simulink model "Joystick_Controller"  (R2025b)
settings: Solver=VariableStepAuto  StartTime=0.0  StopTime=inf  RelTol=1e-3
undefined symbols (not defined in the file): battery_voltage, force_table, pwm_list, voltage_list
libraries: ros2lib x3
settings Model: Creator=vulcangrip  LastModifiedBy=vulcangrip

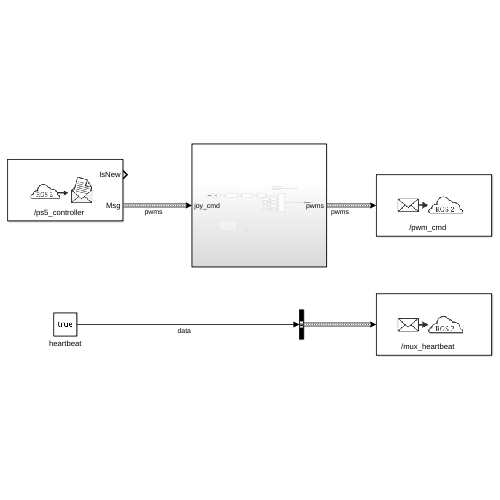
[thumbnail: Simulink's stored preview of the top-level diagram]
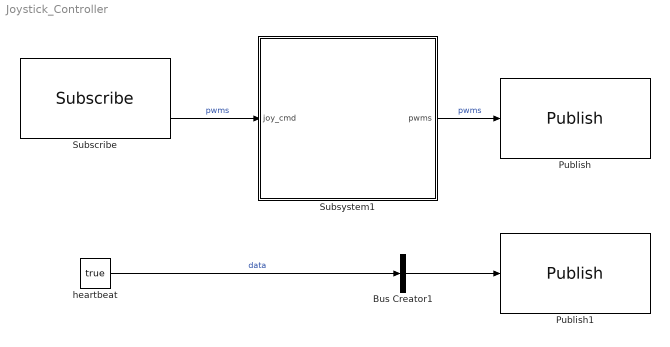
== system Joystick_Controller ==
  Bus Creator1 : BusCreator  Inputs=1  OutDataTypeStr=Bus: SL_Bus_std_msgs_Bool  NonVirtualBus=on
  Publish : ros2lib/Publish  topicSource=Specify your own  topic=/pwm_cmd  messageType=custom_interfaces/Pwms  QOSHistory=Keep last  QOSDepth=10  QOSReliability=Reliable  QOSDurability=Volatile  QOSDeadline=Inf  QOSLifespan=Inf  QOSLiveliness=Automatic  QOSLeaseDuration=Inf  QOSAvoidROSNamespaceConventions=off
  Publish1 : ros2lib/Publish  topicSource=Specify your own  topic=/mux_heartbeat  messageType=std_msgs/Bool  QOSHistory=Keep last  QOSDepth=10  QOSReliability=Reliable  QOSDurability=Volatile  QOSDeadline=Inf  QOSLifespan=Inf  QOSLiveliness=Automatic  QOSLeaseDuration=Inf  QOSAvoidROSNamespaceConventions=off
  Subscribe : ros2lib/Subscribe  topicSource=Specify your own  topic=/ps5_controller  messageType=remote_control_interface/Gamepad  sampleTime=1/60  QOSHistory=Keep last  QOSDepth=10  QOSReliability=Reliable  QOSDurability=Volatile  QOSDeadline=Inf  QOSLifespan=Inf  QOSLiveliness=Automatic  QOSLeaseDuration=Inf  QOSAvoidROSNamespaceConventions=off
  Subsystem1 : Subsystem
  heartbeat : Constant  Value=true
  wires:
  Bus Creator1/1 -> Publish1/1
  heartbeat/1 -> Bus Creator1/1  "data"
  Subscribe/2 -> Subsystem1/1(joy_cmd)  "pwms"
  Subsystem1/1(pwms) -> Publish/1  "pwms"

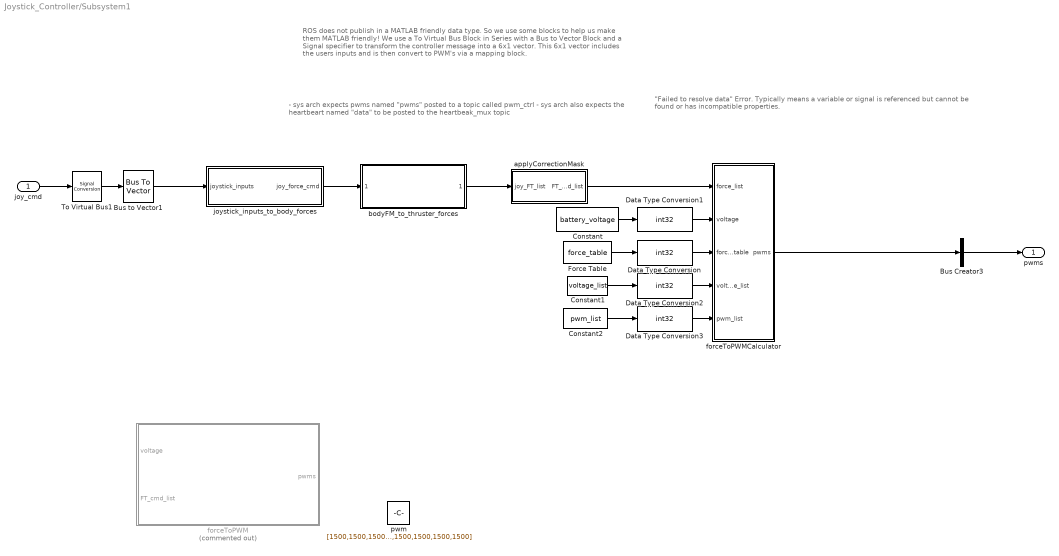
== system Joystick_Controller/Subsystem1 ==
  note: "Failed to resolve data" Error.
      |
      | Typically means a variable or signal is referenced but cannot be found or has incompatible properties.
  note: ROS does not publish in a MATLAB friendly data type. So we use some blocks to help us make them MATLAB friendly!
      |
      | We use a To Virtual Bus Block in Series with a Bus to Vector Block and a Signal specifier to transform the controller message into a 6x1 vector. This 6x1 vector includes the users inputs and is then convert to PWM's via a mapping block.
  note: - sys arch expects pwms named "pwms" posted to a topic called pwm_ctrl
      | - sys arch also expects the heartbeart  named "data" to be posted to the heartbeak_mux topic
  joy_cmd : Inport
  Bus Creator3 : BusCreator  Inputs=1  OutDataTypeStr=Bus: SL_Bus_custom_interfaces_Pwms  NonVirtualBus=on
  Bus to Vector1 : BusToVector
  Constant : Constant  Value=battery_voltage  OutDataTypeStr=int32
  Constant1 : Constant  Value=voltage_list  OutDataTypeStr=int32
  Constant2 : Constant  Value=pwm_list  OutDataTypeStr=int32
  Data Type Conversion{,1..3} (4 alike) : DataTypeConversion  OutDataTypeStr=int32  SaturateOnIntegerOverflow=off  RndMeth=Floor
  Force Table : Constant  Value=force_table  OutDataTypeStr=int32
  To Virtual Bus1 : SignalConversion  ConversionOutput=Virtual bus  OverrideOpt=off
  applyCorrectionMask : Subsystem
  bodyFM_to_thruster_forces : Subsystem  ReferencedSubsystem=bodyFM_to_thruster_forces
  forceToPWM : Subsystem  Commented=on
  forceToPWMCalculator : MATLAB Function  TreatAsAtomicUnit=on
  joystick_inputs_to_body_forces : MATLAB Function  TreatAsAtomicUnit=on
  pwm : Constant  Value=[1500,1500,1500,1500,1500,1500,1500,1500]  OutDataTypeStr=int32
  pwms : Outport
  wires:
  joy_cmd/1 -> To Virtual Bus1/1
  To Virtual Bus1/1 -> Bus to Vector1/1
  Bus to Vector1/1 -> joystick_inputs_to_body_forces/1(joystick_inputs)
  joystick_inputs_to_body_forces/1(joy_force_cmd) -> bodyFM_to_thruster_forces/1
  Bus Creator3/1 -> pwms/1
  bodyFM_to_thruster_forces/1 -> applyCorrectionMask/1(joy_FT_list)
  Constant2/1 -> Data Type Conversion3/1
  Constant/1 -> Data Type Conversion1/1
  Force Table/1 -> Data Type Conversion/1
  Constant1/1 -> Data Type Conversion2/1
  forceToPWMCalculator/1(pwms) -> Bus Creator3/1
  applyCorrectionMask/1(FT_cmd_list) -> forceToPWMCalculator/1(force_list)
  Data Type Conversion1/1 -> forceToPWMCalculator/2(voltage)
  Data Type Conversion/1 -> forceToPWMCalculator/3(force_table)
  Data Type Conversion2/1 -> forceToPWMCalculator/4(voltage_list)
  Data Type Conversion3/1 -> forceToPWMCalculator/5(pwm_list)

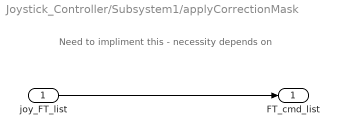
== system Joystick_Controller/Subsystem1/applyCorrectionMask ==
  note: Need to impliment this - necessity depends on
  joy_FT_list : Inport
  FT_cmd_list : Outport
  wires:
  joy_FT_list/1 -> FT_cmd_list/1

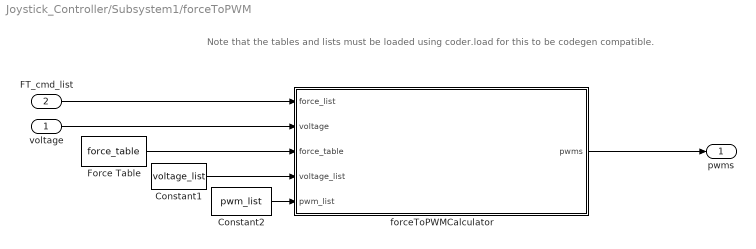
== system Joystick_Controller/Subsystem1/forceToPWM ==
  note: Note that the tables and lists must be loaded using coder.load for this to be codegen compatible.
  voltage : Inport
  FT_cmd_list : Inport  Port=2
  Constant1 : Constant  Value=voltage_list
  Constant2 : Constant  Value=pwm_list
  Force Table : Constant  Value=force_table
  forceToPWMCalculator : MATLAB Function  TreatAsAtomicUnit=on
  pwms : Outport
  wires:
  voltage/1 -> forceToPWMCalculator/2(voltage)
  Constant1/1 -> forceToPWMCalculator/4(voltage_list)
  Constant2/1 -> forceToPWMCalculator/5(pwm_list)
  Force Table/1 -> forceToPWMCalculator/3(force_table)
  FT_cmd_list/1 -> forceToPWMCalculator/1(force_list)
  forceToPWMCalculator/1(pwms) -> pwms/1

== matlab function Joystick_Controller/Subsystem1/forceToPWM/forceToPWMCalculator ==
  data: force_list input; voltage input; pwms output; force_table input; voltage_list input; pwm_list input
function pwms = fcn(force_list,voltage,force_table,voltage_list,pwm_list)

pwms = int32([1500,1500,1500,1500,1500,1500,1500,1500]);

== matlab function Joystick_Controller/Subsystem1/forceToPWMCalculator ==
  data: force_list input; voltage input; pwms output; force_table input; voltage_list input; pwm_list input
function pwms = forceToPWMCalculator(force_list,voltage,force_table,voltage_list,pwm_list)

%pwms = int32(force_list*battery_voltage);
%{
This function figures out what pwm to send in order to get the appropriate
force at the current voltage.


%}
pwms = int32(zeros(size(force_list)));

for k = 1:length(force_list)
    force = force_list(k);

    if(abs(force)<1e-3)
        %if the force setting is very low, just set thruster to stop
        %condition
        pwm_cmd = int32(1500);
    else
        
        %find the closest voltage less than the input voltage
        [~,closest_index] = min(abs(voltage_list-voltage));
       
        %see if the closest_voltage is above or below the input voltage
        if(closest_index==int32(1))
            %no need to do any interpolation, just take the first column for forces
            lower_voltage_index = int32(1);
            upper_voltage_index = int32(1);
    
        elseif(closest_index==length(voltage_list))
            %no need to do any interpolation, just take the last column for forces
            lower_voltage_index = int32(length(voltage_list));
            upper_voltage_index = int32(length(voltage_list));
        elseif(voltage_list(closest_index) < voltage)
            lower_voltage_index = int32(closest_index);
            upper_voltage_index = int32(closest_index+1);
        else
            upper_voltage_index = int32(closest_index);
            lower_voltage_index = int32(closest_index-1);
        end
        
        %average the force column between the two indices\
        if(upper_voltage_index == lower_voltage_index)
            force_column = force_table(lower_voltage_index);
        else
            force_column = force_table(:,lower_voltage_index) + (voltage-voltage_list(lower_voltage_index))*(force_table(:,upper_voltage_index)-force_table(:,lower_voltage_index))/(voltage_list(upper_voltage_index)-voltage_list(lower_voltage_index));
        end
    
        %find the force closest to the input force
        [~,closest_index] = min(abs(force_column-force));
        
        %see if the closest_force is above or below the input force
        if(closest_index==int32(1))
            %no need to do any interpolation, just take the first column for forces
            lower_force_index = int32(1);
            upper_force_index = int32(1);
        elseif(closest_index==length(force_list))
            %no need to do any interpolation, just take the last column for forces
            lower_force_index = int32(length(force_list));
            upper_force_index = int32(length(force_list));
        elseif(force_column(closest_index) < force)
            lower_force_index = int32(closest_index);
            upper_force_index = int32(closest_index+1);
        else
            upper_force_index = int32(closest_index);
            lower_force_index = int32(closest_index-1);
        end
        
        %compute scaling coefficient between neighboring forces
        if(lower_force_index == upper_force_index)
            alpha = int32(0);
        else
            alpha = (force - force_column(upper_force_index))/(force_column(upper_force_index)-force_column(lower_force_index));
        end
    
        %find closest pwm to this force
        pwm_cmd = pwm_list(lower_force_index) + alpha*(pwm_list(upper_force_index)-pwm_list(lower_force_index));
        pwm_cmd = round(pwm_cmd); %round to the nearest integer
    end
    pwms(k) = pwm_cmd;
end

== matlab function Joystick_Controller/Subsystem1/joystick_inputs_to_body_forces ==
  data: joystick_inputs input; joy_force_cmd output
function joy_force_cmd = fcn(joystick_inputs)

%Create the mapping here for PWM values.
%Recall that PWM 1-8 correspond to thruster postions which follow,

%pwm of each thruster on the robot
%In left to right:
%f = front / r = rear
%l = left  / r = right
%t = top   / b = bottom
%PWM(1)=pwm_flt
%PWM(2)=pwm_frt
%PWM(3)=pwm_rlt
%PWM(4)=pwm_rrt
%PWM(5)=pwm_flb
%PWM(6)=pwm_frb
%PWM(7)=pwm_rlb
%PWM(8)=pwm_rrb

%unpacking joystick inputs
x = joystick_inputs(1);
y = joystick_inputs(2);
pitch = joystick_inputs(3);
yaw = joystick_inputs(4);
sink = joystick_inputs(5);
rise = joystick_inputs(6);




force = [ x y 0 0 pitch yaw];


force(1) = sin(x);

force(2) = cos(y);

force(5) = sin(pitch);

force(6) = cos(yaw);

if sink == rise
    force(3) = 0;

else 
    force(3) = rise - sink;
end

joy_force_cmd = int32(joystick_inputs+1);

%Need to specify int32 for the output data type to maintain consistent
